simulink model "sldemo_mdlref_variants"  (Simulink 10.0)
settings: Solver=FixedStepDiscrete  StartTime=0.0  StopTime=10.0  RelTol=1e-3  EnableMultiTasking=on
PreLoadFcn:
  | V_LINEAR_CONTROLLER=Simulink.Variant('CTRL==1');
  | V_NONLINEAR_CONTROLLER=Simulink.Variant('CTRL==2');
  | 
  | CTRL=2;
Description:
  | Model Reference Variants
  | 
  | This demo illustrates model reference variants. A Model block is used to
  | reference one Simulink(R) model from another Simulink model. A Model block can
  | have different variants. A variant describes one of N possible modes a Model
  | block can operate in. Each variant of the Model block references a specific
  | model with model specific arguments. Only one variant is active for
  | simulation. You can switch the active variant of a Model block by changing the
  | values of variables in the base workspace or manually overriding variant
  | selection using the Model block dialog.
CloseFcn:
  | clear CTRL V_LINEAR_CONTROLLER V_NONLINEAR_CONTROLLER;
settings Model: Creator=The MathWorks, Inc.  ModifiedByFormat=The MathWorks Inc.  LastModifiedBy=The MathWorks Inc.
settings DataIOCC: LimitDataPoints=on  SaveTime=off
settings OptimizationCC: DefaultParameterBehavior=Inlined  ExpressionDepthLimit=2147483647
settings DebuggingCC: UnderspecifiedInitializationDetection=Simplified  MergeDetectMultiDrivingBlocksExec=error  SolverPrmCheckMsg=warning  FcnCallInpInsideContextMsg=warning  StateNameClashWarn=warning
settings GRTTargetCC: GeneratePreprocessorConditionals=Disable all
settings ConfigComp: CovExternalEMLEnable=off  CovSFcnEnable=off

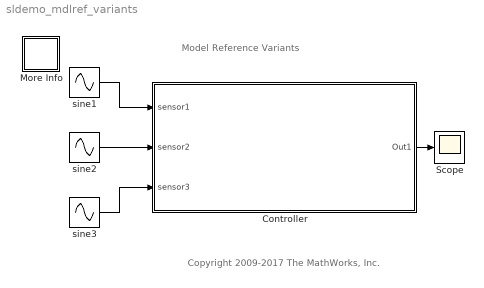
== system sldemo_mdlref_variants ==
  note: Copyright 2009-2017 The MathWorks, Inc.
  note: Model Reference Variants
  Controller : Subsystem  Variant=on
      settings: GeneratePreprocessorConditionals=on
  More Info : Subsystem
      settings: OpenFcn=showdemo(bdroot(gcb))
      mask Display: disp('?')
  Scope : Scope
  sine1 : Sin  Amplitude=.1  Frequency=pi/3  SampleTime=.01
  sine2 : Sin  Amplitude=2  SampleTime=.01
  sine3 : Sin  Amplitude=.3  Frequency=pi/6  SampleTime=.01
  wires:
  sine1/1 -> Controller/1("sensor1 ")
  sine2/1 -> Controller/2("sensor2 ")
  sine3/1 -> Controller/3("sensor3 ")
  Controller/1(" Out1") -> Scope/1

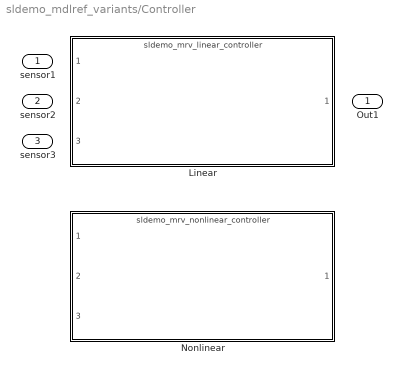
== system sldemo_mdlref_variants/Controller ==
  "sensor1 " : Inport
  "sensor2 " : Inport  Port=2
  "sensor3 " : Inport  Port=3
  Linear : ModelReference  ModelNameDialog=sldemo_mrv_linear_controller  SimulationMode=Normal  VariantControl=V_LINEAR_CONTROLLER  ModelReferenceVersion=1.17
  Nonlinear : ModelReference  ModelNameDialog=sldemo_mrv_nonlinear_controller  SimulationMode=Normal  VariantControl=V_NONLINEAR_CONTROLLER  ModelReferenceVersion=1.18
  " Out1" : Outport  VectorParamsAs1DForOutWhenUnconnected=off

== system sldemo_mdlref_variants/More Info ==
  note: This demo illustrates model reference variants. A Model block is used to
      | reference one Simulink model from another Simulink model. A Model block can
      | have different variants. A variant describes one of N possible modes a Model
      | block can operate in. Each variant of the Model block references a specific
      | model with model specific arguments. Only one variant is active for
      | simulation. You can switch the active variant of a Model block by changing the
      | values of variables in the base workspace or manually overriding variant
      | selection using the Model block dialog.
  note: Model Reference Variants
